simulink model "PMSM_VF"  (R2022a)
settings: Solver=FixedStepAuto  StartTime=0.0  StopTime=10  FixedStep=Ts  RelTol=1e-3  EnableMultiTasking=on
values from neighbouring files (symbols this model uses):
  Ts = T_pwm    (= 5e-05)    [BR2804_1700Kv.m]
  Vmin = 1    [BR2804_1700Kv.m]
undefined symbols (not defined in the file or in its folder): pmsm
libraries: simulink x2, eeGeneralControl x2, eeTransforms x2, mcbplantlib x1, autolibpmsmexterior x1
settings Model: Creator=徐国强  LastModifiedBy=徐国强
settings SolverCC: AutoInsertRateTranBlk=on
settings OptimizationCC: DefaultParameterBehavior=Inlined  EnhancedBackFolding=on  PassReuseOutputArgsAs=Individual arguments  ZeroExternalMemoryAtStartup=off  ZeroInternalMemoryAtStartup=off  OptimizeBlockOrder=speed  DifferentSizesBufferReuse=on  OptimizationCustomize=off  EfficientTunableParamExpr=on
settings DebuggingCC: ParameterTunabilityLossMsg=error
settings HardwareCC: ProdBitPerPointer=32  ProdBitPerSizeT=32  ProdBitPerPtrDiffT=32  ProdLargestAtomicInteger=Long  ProdLargestAtomicFloat=Double  ProdWordSize=32  ProdHWDeviceType=ARM Compatible->ARM Cortex-M
settings SFSimCC: MATLABDynamicMemAlloc=off
settings RTWCC: SystemTargetFile=ert.tlc  GenCodeOnly=on  TemplateMakefile=ert_default_tmf  GenerateReport=on  LaunchReport=on
settings CodeAppCC: ForceParamTrailComments=on  IgnoreCustomStorageClasses=off  OperatorAnnotations=on  SimulinkDataObjDesc=on  SFDataObjDesc=on  InsertBlockDesc=on
settings ERTTargetCC: TargetLangStandard=C99 (ISO)  InlinedParameterPlacement=NonHierarchical  ERTCustomFileTemplate=example_file_process.tlc

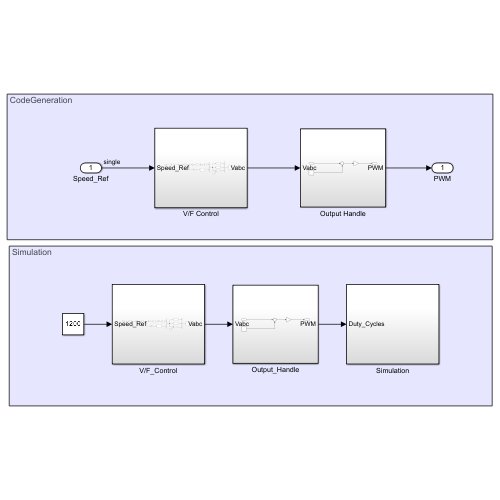
[thumbnail: Simulink's stored preview of the top-level diagram]
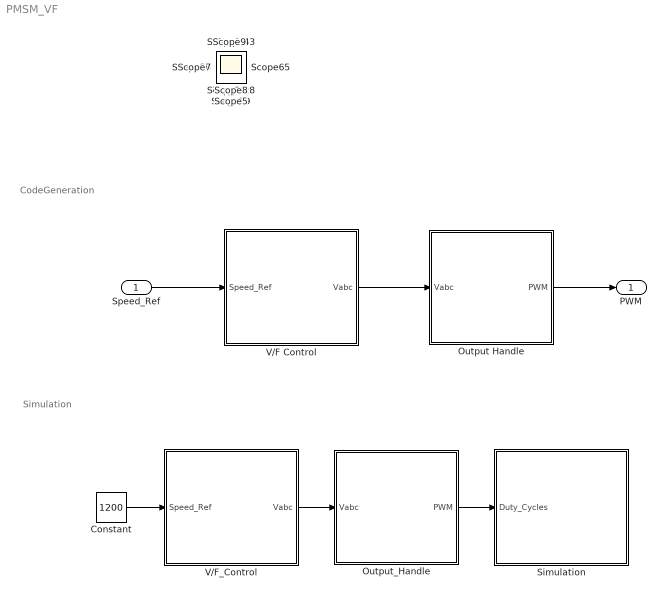
== system PMSM_VF ==
  note: CodeGeneration
  note: Simulation
  Speed_Ref : Inport  OutDataTypeStr=single
  Constant : Constant  Value=1200  OutDataTypeStr=single
  Output Handle : Subsystem
  Output_Handle : Subsystem
  Simulation : Subsystem
  V/F Control : Subsystem
  V/F_Control : Subsystem
  PWM : Outport
  Scope{,1..31} (32 alike) : Scope
  wires:
  V/F Control/1(Vabc) -> Output Handle/1(Vabc)
  V/F_Control/1(Vabc) -> Output_Handle/1(Vabc)
  Output_Handle/1(PWM) -> Simulation/1(Duty_Cycles)
  Constant/1 -> V/F_Control/1(Speed_Ref)
  Speed_Ref/1 -> V/F Control/1(Speed_Ref)
  Output Handle/1(PWM) -> PWM/1

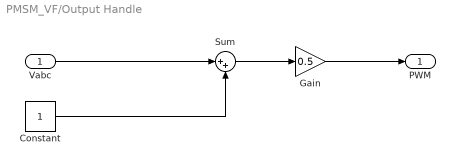
== system PMSM_VF/Output Handle ==
  Vabc : Inport
  Constant : Constant  OutDataTypeStr=single
  Gain : Gain  Gain=0.5
  Sum : Sum  Inputs=|++
  PWM : Outport
  wires:
  Constant/1 -> Sum/2
  Vabc/1 -> Sum/1
  Sum/1 -> Gain/1
  Gain/1 -> PWM/1

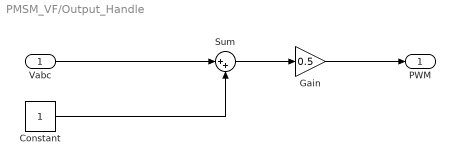
== system PMSM_VF/Output_Handle ==
  Vabc : Inport
  Constant : Constant  OutDataTypeStr=single
  Gain : Gain  Gain=0.5
  Sum : Sum  Inputs=|++
  PWM : Outport
  wires:
  Constant/1 -> Sum/2
  Vabc/1 -> Sum/1
  Sum/1 -> Gain/1
  Gain/1 -> PWM/1

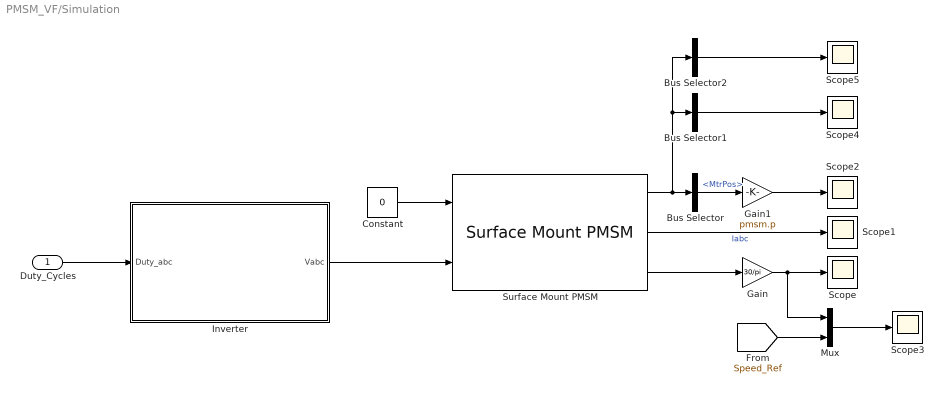
== system PMSM_VF/Simulation ==
  Duty_Cycles : Inport
  Bus Selector : BusSelector  OutputSignals=MtrPos
  Bus Selector1 : BusSelector  OutputSignals=IdSync,IqSync  OutputAsBus=on
  Bus Selector2 : BusSelector  OutputSignals=MtrTrq  OutputAsBus=on
  Constant : Constant  Value=0
  Gain : Gain  Gain=30/pi  OutDataTypeStr=single
  Gain1 : Gain  Gain=pmsm.p
  Inverter : Subsystem
  Mux : Mux  Inputs=2
  Scope{,1..5} (6 alike) : Scope
  Surface Mount PMSM : autolibpmsmexterior/Surface Mount PMSM  port_config=Torque  sim_type=Discrete  Ts=Ts  P=pmsm.p  Rs=pmsm.Rs  Ldq_=pmsm.Ld  KConstText=Permanent flux linkage constant (lambda_pm):  lambda_pm=pmsm.FluxPM  Ke=159.9771  Kt=1.323  mechanical=[pmsm.J, pmsm.B, 0]  idq0=[0 0]  theta_init=0  omega_init=0  KConst=pmsm.FluxPM  lambda_pm_calc=pmsm.FluxPM  RefBlkName='autolibpmsmexterior/Surface Mount PMSM'  aMode=5  Ldq="[0.0006      0.0006]"
      settings: SourceProductBaseCode=PW,DR,MT,VE
  wires:
  Inverter/1(Vabc) -> Surface Mount PMSM/2
  Duty_Cycles/1 -> Inverter/1(Duty_abc)
  Surface Mount PMSM/3 -> Gain/1
  Gain/1 -> Mux/1, Scope/1
  Surface Mount PMSM/2 -> Scope1/1  "Iabc"
  Surface Mount PMSM/1 -> Bus Selector2/1, Bus Selector1/1, Bus Selector/1
  Bus Selector/1 -> Gain1/1  "<MtrPos>"
  Gain1/1 -> Scope2/1
  Constant/1 -> Surface Mount PMSM/1
  [Speed_Ref] -> Mux/2
  Mux/1 -> Scope3/1
  Bus Selector1/1 -> Scope4/1
  Bus Selector2/1 -> Scope5/1

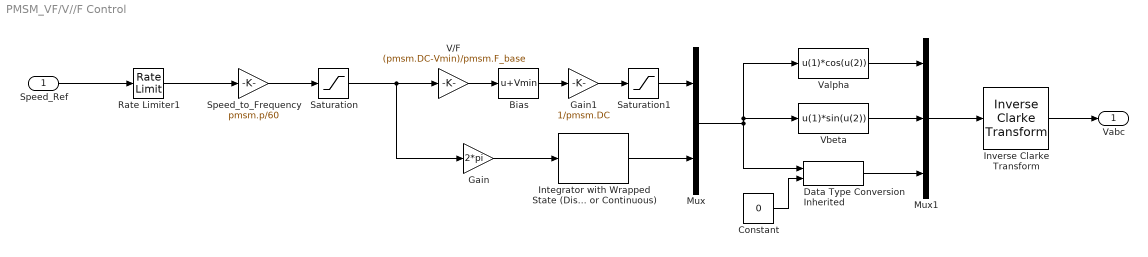
== system PMSM_VF/V//F Control ==
  Speed_Ref : Inport
  Bias : Bias  Bias=Vmin  SaturateOnIntegerOverflow=off
  Constant : Constant  Value=0  OutDataTypeStr=single
  Data Type Conversion Inherited : simulink/Signal Attributes/Data Type Conversion Inherited  ConvertRealWorld=Real World Value  DoSatur=off
      settings: SourceProductBaseCode=SL
  Gain : Gain  Gain=2*pi
  Gain1 : Gain  Gain=1/pmsm.DC
  Integrator with Wrapped State (Discrete or Continuous) : eeGeneralControl/Integrator with Wrapped State (Discrete or Continuous)  LabelModeActiveChoice=Discrete  WrappedStateUpperValue=2*pi  WrappedStateLowerValue=0  x0=0  Ts=Ts
      settings: SourceProductBaseCode=PS
  Inverse Clarke Transform : eeTransforms/Inverse Clarke Transform  PowerInvariant=off
      settings: SourceProductBaseCode=PS
  Mux : Mux  Inputs=2
  Mux1 : Mux  Inputs=3
  Rate Limiter1 : RateLimiter  RisingSlewLimit=500  FallingSlewLimit=-500  SampleTimeMode=inherited
  Saturation : Saturate  UpperLimit=pmsm.F_base  LowerLimit=0
  Saturation1 : Saturate  UpperLimit=1  LowerLimit=0
  Speed_to_Frequency : Gain  Gain=pmsm.p/60
  V/F : Gain  Gain=(pmsm.DC-Vmin)/pmsm.F_base
  Valpha : Fcn  Expr=u(1)*cos(u(2))
  Vbeta : Fcn  Expr=u(1)*sin(u(2))
  Vabc : Outport
  wires:
  Speed_Ref/1 -> Rate Limiter1/1
  Rate Limiter1/1 -> Speed_to_Frequency/1
  Speed_to_Frequency/1 -> Saturation/1
  Saturation/1 -> Gain/1, V/F/1
  V/F/1 -> Bias/1
  Gain/1 -> Integrator with Wrapped State (Discrete or Continuous)/1
  Integrator with Wrapped State (Discrete or Continuous)/1 -> Mux/2
  Mux/1 -> Vbeta/1, Valpha/1, Data Type Conversion Inherited/1
  Vbeta/1 -> Mux1/2
  Valpha/1 -> Mux1/1
  Mux1/1 -> Inverse Clarke Transform/1
  Bias/1 -> Gain1/1
  Gain1/1 -> Saturation1/1
  Saturation1/1 -> Mux/1
  Inverse Clarke Transform/1 -> Vabc/1
  Data Type Conversion Inherited/1 -> Mux1/3
  Constant/1 -> Data Type Conversion Inherited/2

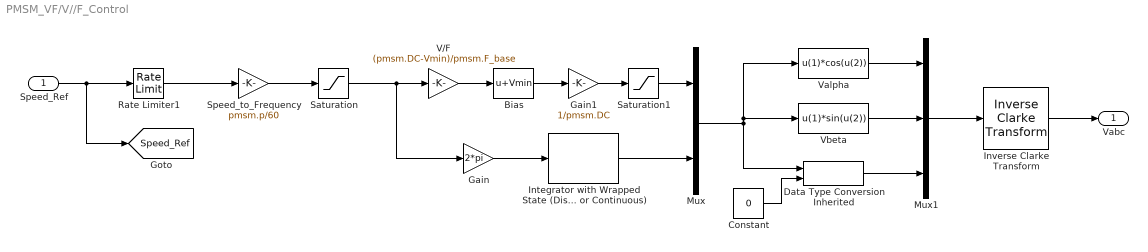
== system PMSM_VF/V//F_Control ==
  Speed_Ref : Inport
  Bias : Bias  Bias=Vmin  SaturateOnIntegerOverflow=off
  Constant : Constant  Value=0  SampleTime=Ts
  Data Type Conversion Inherited : simulink/Signal Attributes/Data Type Conversion Inherited  ConvertRealWorld=Real World Value  DoSatur=off
      settings: SourceProductBaseCode=SL
  Gain : Gain  Gain=2*pi
  Gain1 : Gain  Gain=1/pmsm.DC
  Integrator with Wrapped State (Discrete or Continuous) : eeGeneralControl/Integrator with Wrapped State (Discrete or Continuous)  LabelModeActiveChoice=Discrete  WrappedStateUpperValue=2*pi  WrappedStateLowerValue=0  x0=0  Ts=Ts
      settings: SourceProductBaseCode=PS
  Inverse Clarke Transform : eeTransforms/Inverse Clarke Transform  PowerInvariant=off
      settings: SourceProductBaseCode=PS
  Mux : Mux  Inputs=2
  Mux1 : Mux  Inputs=3
  Rate Limiter1 : RateLimiter  RisingSlewLimit=500  FallingSlewLimit=-500  SampleTimeMode=inherited
  Saturation : Saturate  UpperLimit=pmsm.F_base  LowerLimit=0
  Saturation1 : Saturate  UpperLimit=1  LowerLimit=0
  Speed_to_Frequency : Gain  Gain=pmsm.p/60
  V/F : Gain  Gain=(pmsm.DC-Vmin)/pmsm.F_base
  Valpha : Fcn  Expr=u(1)*cos(u(2))
  Vbeta : Fcn  Expr=u(1)*sin(u(2))
  Vabc : Outport
  tag scope: Speed_Ref=global
  wires:
  Speed_Ref/1 -> [Speed_Ref], Rate Limiter1/1
  Rate Limiter1/1 -> Speed_to_Frequency/1
  Speed_to_Frequency/1 -> Saturation/1
  Saturation/1 -> Gain/1, V/F/1
  V/F/1 -> Bias/1
  Gain/1 -> Integrator with Wrapped State (Discrete or Continuous)/1
  Integrator with Wrapped State (Discrete or Continuous)/1 -> Mux/2
  Mux/1 -> Vbeta/1, Valpha/1, Data Type Conversion Inherited/1
  Constant/1 -> Data Type Conversion Inherited/2
  Vbeta/1 -> Mux1/2
  Valpha/1 -> Mux1/1
  Data Type Conversion Inherited/1 -> Mux1/3
  Mux1/1 -> Inverse Clarke Transform/1
  Bias/1 -> Gain1/1
  Gain1/1 -> Saturation1/1
  Saturation1/1 -> Mux/1
  Inverse Clarke Transform/1 -> Vabc/1

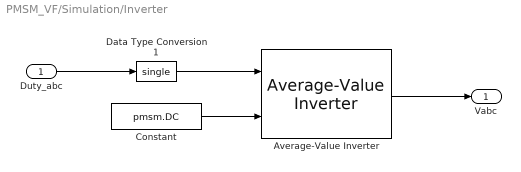
== system PMSM_VF/Simulation/Inverter ==
  Duty_abc : Inport
  Average-Value Inverter : mcbplantlib/Average-Value Inverter
  Constant : Constant  Value=pmsm.DC  OutDataTypeStr=single
  Data Type Conversion1 : DataTypeConversion  OutDataTypeStr=single  RndMeth=Simplest  SaturateOnIntegerOverflow=off
  Vabc : Outport  VectorParamsAs1DForOutWhenUnconnected=off
  wires:
  Duty_abc/1 -> Data Type Conversion1/1
  Data Type Conversion1/1 -> Average-Value Inverter/1
  Average-Value Inverter/1 -> Vabc/1
  Constant/1 -> Average-Value Inverter/2
